simulink model "GFLIB_ControllerPIpAW_BAM_F16"  (Simulink 8.3)
settings: Solver=ode45  StartTime=0.0  StopTime=10.0  RelTol=1e-3
undefined symbols (not defined in the file): f16IntegGain, f16PropGain, s16IntegGainShift, s16PropGainShift
settings Model: Creator=B17364  LastModifiedBy=B17364
settings DataIOCC: SignalLoggingSaveFormat=Dataset
settings DebuggingCC: UnderspecifiedInitializationDetection=Simplified  StateNameClashWarn=none
settings GRTTargetCC: CombineOutputUpdateFcns=on  GRTInterface=off

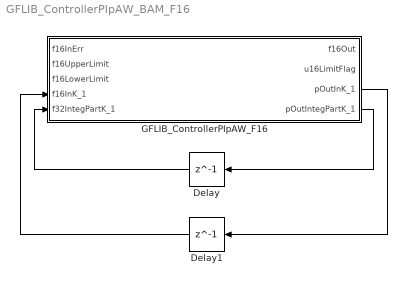
== system GFLIB_ControllerPIpAW_BAM_F16 ==
  Delay : Delay  DelayLength=1  InitialCondition=0
  Delay1 : Delay  DelayLength=1  InitialCondition=0
  GFLIB_ControllerPIpAW_F16 : Subsystem  mask(GFLIB_ControllerPIpAW_F16){f16PropGain=f16PropGain, s16PropGainShift=s16PropGainShift, f16IntegGain=f16IntegGain, s16IntegGainShift=s16IntegGainShift}
      mask help: Bit accurate model of parallel form PI controller with anti-windup. All parameters as well as input and output are 16-bit integers except for u16NShift parameter which is 16-bit unsigned integer.
      mask init:
      | pos = get_param(gcb, 'Position');width = pos(3) - pos(1); height = pos(4) - pos(2);tX=width/2;tY=height*0.9;
      mask Display: color('black');port_label('input',1,'f16InErr');port_label('input',2,'f16UpperLimit');port_label('input',3,'f16LowerLimit');port_label('input',4,'f16InK_1');port_label('input',5,'f32IntegPartK_1');port_label('output',1,'f16Out');port_label('output',2,'u16LimitFlag');port_label('output',3,'pOutInK_1');port_label('output',4,'pOutIntegPartK_1');color('black');disp('GFLIB_ControllerPIpAW_F16');color('blue');text(tX,tY, 'BAM', 'horizontalAlignment', 'center');
  wires:
  GFLIB_ControllerPIpAW_F16/4(pOutIntegPartK_1) -> Delay/1
  GFLIB_ControllerPIpAW_F16/3(pOutInK_1) -> Delay1/1
  Delay/1 -> GFLIB_ControllerPIpAW_F16/5(f32IntegPartK_1)
  Delay1/1 -> GFLIB_ControllerPIpAW_F16/4(f16InK_1)

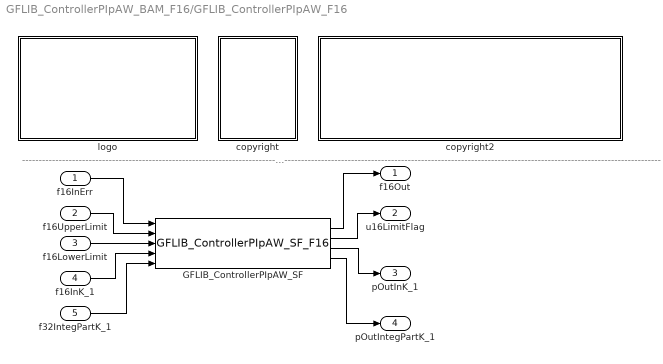
== system GFLIB_ControllerPIpAW_BAM_F16/GFLIB_ControllerPIpAW_F16 ==
  note: ---------------------------------------------------------------------------------------------------------------------------------------------------------------------------------------------------
  f16InErr : Inport
  f16UpperLimit : Inport  Port=2
  f16LowerLimit : Inport  Port=3
  f16InK_1 : Inport  Port=4
  f32IntegPartK_1 : Inport  Port=5
  GFLIB_ControllerPIpAW_SF : S-Function  FunctionName=GFLIB_ControllerPIpAW_SF_F16  Parameters=f16PropGain,s16PropGainShift,f16IntegGain,s16IntegGainShift  EnableBusSupport=off
  copyright : Subsystem
      mask Display: text(10,90,'FILE:');text(10,75,'DESRIPTION:');text(10,60,'COPYRIGHT:');text(10,45,'VERSION:');text(10,30,'DATE:')
  copyright2 : Subsystem
      mask Display: text(10,90,'GFLIB_ControllerPIpAW_BAM_F16.mdl');text(10,75,'Parallel form of a standard PI controller with implemented anti-windup.');text(10,60,'Freescale');text(10,45,'0.1');text(10,30,'12-Jun-2015');
  logo : Subsystem
      mask Display: image(imread('logo.jpg'))
  f16Out : Outport
  u16LimitFlag : Outport  Port=2
  pOutInK_1 : Outport  Port=3
  pOutIntegPartK_1 : Outport  Port=4
  wires:
  f16InErr/1 -> GFLIB_ControllerPIpAW_SF/1
  f16UpperLimit/1 -> GFLIB_ControllerPIpAW_SF/2
  f16LowerLimit/1 -> GFLIB_ControllerPIpAW_SF/3
  f16InK_1/1 -> GFLIB_ControllerPIpAW_SF/4
  f32IntegPartK_1/1 -> GFLIB_ControllerPIpAW_SF/5
  GFLIB_ControllerPIpAW_SF/1 -> f16Out/1
  GFLIB_ControllerPIpAW_SF/2 -> u16LimitFlag/1
  GFLIB_ControllerPIpAW_SF/3 -> pOutInK_1/1
  GFLIB_ControllerPIpAW_SF/4 -> pOutIntegPartK_1/1

== system GFLIB_ControllerPIpAW_BAM_F16/GFLIB_ControllerPIpAW_F16/copyright ==

== system GFLIB_ControllerPIpAW_BAM_F16/GFLIB_ControllerPIpAW_F16/copyright2 ==

== system GFLIB_ControllerPIpAW_BAM_F16/GFLIB_ControllerPIpAW_F16/logo ==
